simulink model "SimpleSpringMassSystemModel"  (R2016b)
settings: Solver=ode45  StartTime=0.0  StopTime=50  MaxStep=0.05  RelTol=1e-3
undefined symbols (not defined in the file): b, k, m
settings Model: Creator=shyam  LastModifiedBy=shyam

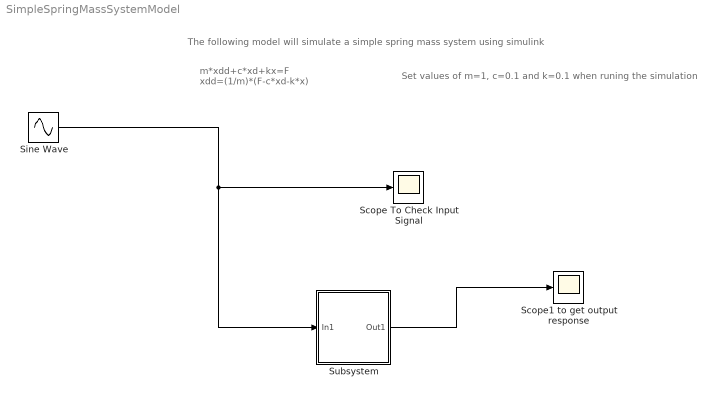
== system SimpleSpringMassSystemModel ==
  note: Set values of m=1, c=0.1 and k=0.1 when runing the simulation
  note: The following model will simulate a simple spring mass system using simulink
  note: m*xdd+c*xd+kx=F
      | xdd=(1/m)*(F-c*xd-k*x)
  "Scope To Check Input Signal " : Scope
  "Scope1 to get output response " : Scope
  Sine Wave : Sin  Amplitude=2  SampleTime=0
  Subsystem : Subsystem
  wires:
  Sine Wave/1 -> Subsystem/1(In1), "Scope To Check Input Signal "/1
  Subsystem/1(Out1) -> "Scope1 to get output response "/1

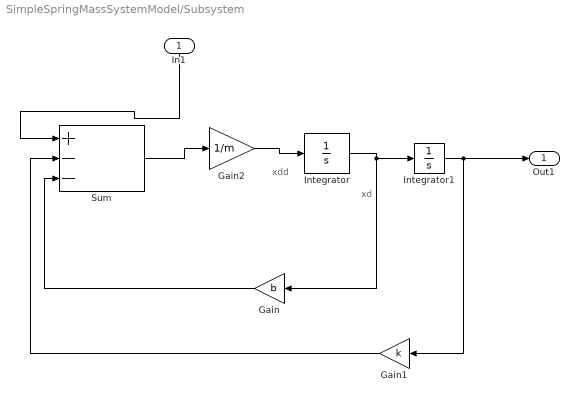
== system SimpleSpringMassSystemModel/Subsystem ==
  note: xdd
  note: xd
  In1 : Inport
  Gain : Gain  Gain=b
  Gain1 : Gain  Gain=k
  Gain2 : Gain  Gain=1/m
  Integrator : Integrator
  Integrator1 : Integrator
  Sum : Sum  Inputs=+--
  Out1 : Outport
  wires:
  In1/1 -> Sum/1
  Sum/1 -> Gain2/1
  Integrator1/1 -> Out1/1, Gain1/1
  Integrator/1 -> Gain/1, Integrator1/1
  Gain2/1 -> Integrator/1
  Gain/1 -> Sum/3
  Gain1/1 -> Sum/2
